simulink model "quadruped_robot_jacobian2"  (R2021a)
settings: Solver=ode15s  StartTime=0.0  StopTime=50  EnableMultiTasking=on
undefined symbols (not defined in the file): C, com_initial_height, H, Kvec, L, L1, L2, L3, leg1, leg2, leg3, leg4, q0, q0_leg1, q0_leg2, q0_leg3, q0_leg4, X, Y, Z
libraries: sm_lib x52, nesl_utility x28, roblocks x8, simulink_extras x1
(part 3 of 3)

== matlab function quadruped_robot_jacobian2/new_recalculate_legs_position ==
  data: u_rpy input; new_leg_pos output; legs_pos input
function new_leg_pos = new_recalculate_legs_position(u_rpy, legs_pos)
% u_rpy = [roll; pitch; yaw]  (rad)
% legs_pos = [x1; y1; z1; x2; …] em frame mundo W

roll  = u_rpy(1);
pitch = u_rpy(2);
yaw = u_rpy(3);

% Matriz que DESinclina
% R_nivel = rotx(rad2deg( roll )) * roty(rad2deg( pitch )); % apenas roll & pitch
R_nivel = rotx(rad2deg( roll )) * roty(rad2deg( pitch )) * rotz(rad2deg( yaw )); % roll, pitch e yaw

new_leg_pos = zeros(12,1);
for k = 1:4
    idx  = 3*(k-1)+(1:3);        % índices 1:3 4:6 …
    v_B = R_nivel' * legs_pos(idx); % remove só roll/pitch
    new_leg_pos(idx) = v_B;  % alvo no mundo
end
end
